simulink model "V2021_M2_P1_P"  (R2021a)
settings: Solver=VariableStepAuto  StartTime=0.0  StopTime=500  RelTol=1e-3
undefined symbols (not defined in the file): f_eff, J_eff, Kb, Ktn, L, Pos_ref, R, time
settings Model: Creator=azzam  LastModifiedBy=azzam
settings DebuggingCC: UnconnectedInputMsg=none  UnconnectedOutputMsg=none  UnconnectedLineMsg=none
settings ModelReferenceCC: EnableRefExpFcnMdlSchedulingChecks=off
settings RTWCC: Description=Generic Real-Time Target  DLArmComputeVersion=20.02.1

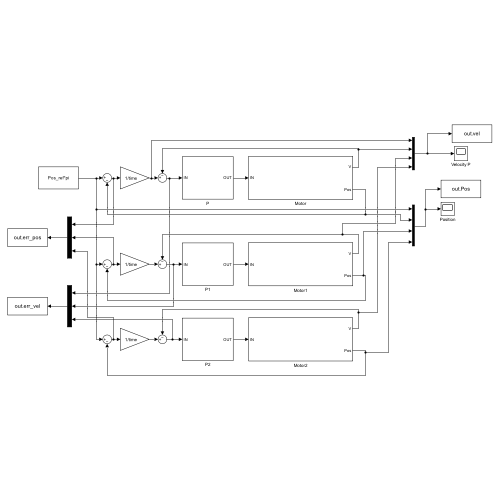
[thumbnail: Simulink's stored preview of the top-level diagram]
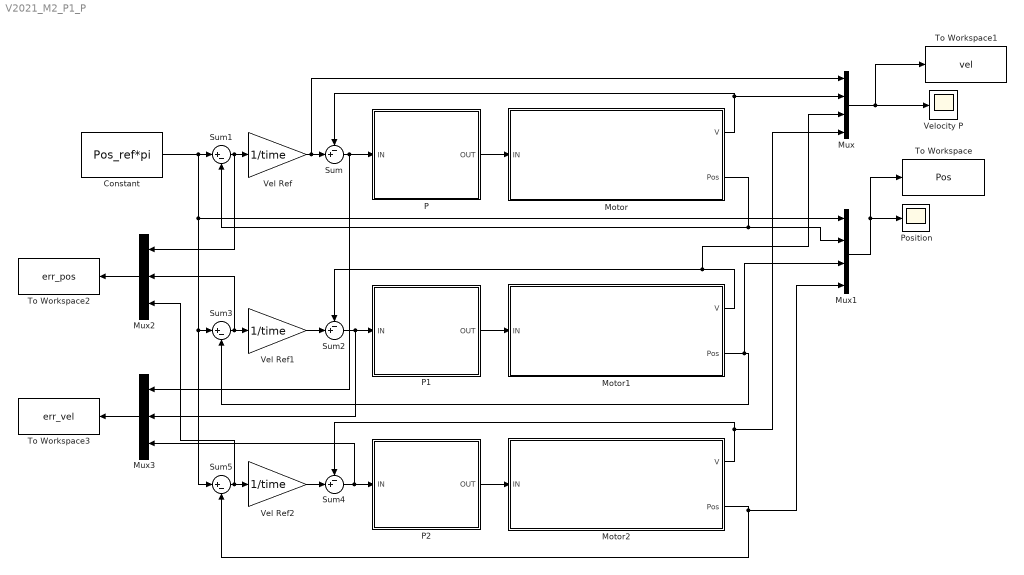
== system V2021_M2_P1_P ==
  Constant : Constant  Value=Pos_ref*pi
  Motor : Subsystem
  Motor1 : Subsystem
  Motor2 : Subsystem
  Mux : Mux
  Mux1 : Mux
  Mux2 : Mux  Inputs=3
  Mux3 : Mux  Inputs=3
  P : Subsystem
  P1 : Subsystem
  P2 : Subsystem
  Position : Scope
  Sum : Sum  Inputs=-+|
  Sum1 : Sum  Inputs=|+-
  Sum2 : Sum  Inputs=-+|
  Sum3 : Sum  Inputs=|+-
  Sum4 : Sum  Inputs=-+|
  Sum5 : Sum  Inputs=|+-
  To Workspace : ToWorkspace  VariableName=Pos  SaveFormat=Timeseries  SampleTime=-1
  To Workspace1 : ToWorkspace  VariableName=vel  SaveFormat=Timeseries  SampleTime=-1
  To Workspace2 : ToWorkspace  VariableName=err_pos  SaveFormat=Timeseries  SampleTime=-1
  To Workspace3 : ToWorkspace  VariableName=err_vel  SaveFormat=Timeseries  SampleTime=-1
  Vel Ref : Gain  Gain=1/time
  Vel Ref1 : Gain  Gain=1/time
  Vel Ref2 : Gain  Gain=1/time
  Velocity P : Scope
  wires:
  Sum/1 -> P/1(IN), Mux3/1
  Sum1/1 -> Mux2/1, Vel Ref/1
  Vel Ref/1 -> Sum/2, Mux/1
  Motor/2(Pos) -> Sum1/2, Mux1/2
  Mux/1 -> To Workspace1/1, Velocity P/1
  Motor/1(V) -> Sum/1, Mux/2
  P/1(OUT) -> Motor/1(IN)
  Mux1/1 -> To Workspace/1, Position/1
  Motor1/2(Pos) -> Mux1/3, Sum3/2
  P1/1(OUT) -> Motor1/1(IN)
  Motor1/1(V) -> Mux/3, Sum2/1
  Sum3/1 -> Mux2/2, Vel Ref1/1
  Sum2/1 -> P1/1(IN), Mux3/2
  Vel Ref1/1 -> Sum2/2
  Constant/1 -> Sum5/1, Sum3/1, Mux1/1, Sum1/1
  Vel Ref2/1 -> Sum4/2
  Motor2/1(V) -> Mux/4, Sum4/1
  Sum4/1 -> P2/1(IN), Mux3/3
  Sum5/1 -> Mux2/3, Vel Ref2/1
  P2/1(OUT) -> Motor2/1(IN)
  Motor2/2(Pos) -> Mux1/4, Sum5/2
  Mux2/1 -> To Workspace2/1
  Mux3/1 -> To Workspace3/1

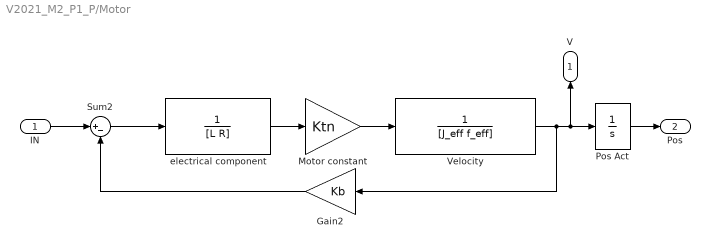
== system V2021_M2_P1_P/Motor ==
  IN : Inport
  Gain2 : Gain  Gain=Kb
  Motor constant : Gain  Gain=Ktn
  Pos Act : Integrator
  Sum2 : Sum  Inputs=|+-
  Velocity : TransferFcn  Denominator=[J_eff f_eff]
  electrical component : TransferFcn  Denominator=[L R]
  V : Outport
  Pos : Outport  Port=2
  wires:
  electrical component/1 -> Motor constant/1
  Motor constant/1 -> Velocity/1
  Sum2/1 -> electrical component/1
  IN/1 -> Sum2/1
  Gain2/1 -> Sum2/2
  Velocity/1 -> V/1, Pos Act/1, Gain2/1
  Pos Act/1 -> Pos/1

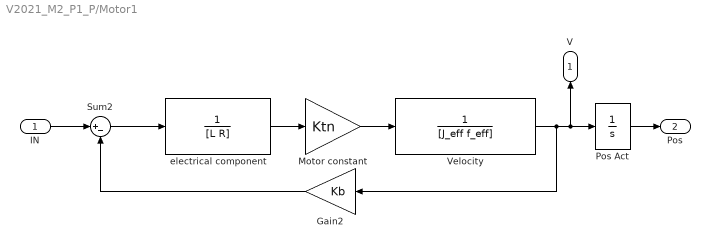
== system V2021_M2_P1_P/Motor1 ==
  IN : Inport
  Gain2 : Gain  Gain=Kb
  Motor constant : Gain  Gain=Ktn
  Pos Act : Integrator
  Sum2 : Sum  Inputs=|+-
  Velocity : TransferFcn  Denominator=[J_eff f_eff]
  electrical component : TransferFcn  Denominator=[L R]
  V : Outport
  Pos : Outport  Port=2
  wires:
  electrical component/1 -> Motor constant/1
  Motor constant/1 -> Velocity/1
  Sum2/1 -> electrical component/1
  IN/1 -> Sum2/1
  Gain2/1 -> Sum2/2
  Velocity/1 -> V/1, Pos Act/1, Gain2/1
  Pos Act/1 -> Pos/1

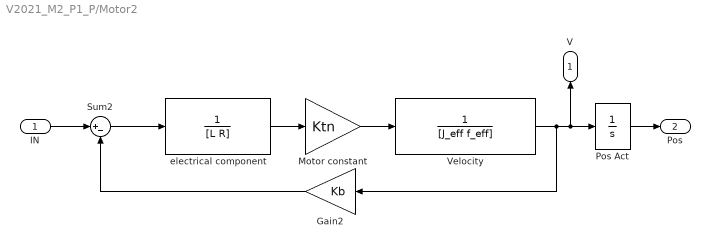
== system V2021_M2_P1_P/Motor2 ==
  IN : Inport
  Gain2 : Gain  Gain=Kb
  Motor constant : Gain  Gain=Ktn
  Pos Act : Integrator
  Sum2 : Sum  Inputs=|+-
  Velocity : TransferFcn  Denominator=[J_eff f_eff]
  electrical component : TransferFcn  Denominator=[L R]
  V : Outport
  Pos : Outport  Port=2
  wires:
  electrical component/1 -> Motor constant/1
  Motor constant/1 -> Velocity/1
  Sum2/1 -> electrical component/1
  IN/1 -> Sum2/1
  Gain2/1 -> Sum2/2
  Velocity/1 -> V/1, Pos Act/1, Gain2/1
  Pos Act/1 -> Pos/1

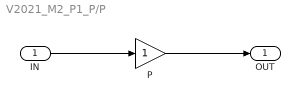
== system V2021_M2_P1_P/P ==
  IN : Inport
  P : Gain
  OUT : Outport
  wires:
  IN/1 -> P/1
  P/1 -> OUT/1

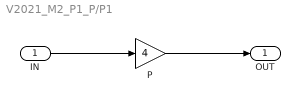
== system V2021_M2_P1_P/P1 ==
  IN : Inport
  P : Gain  Gain=4
  OUT : Outport
  wires:
  P/1 -> OUT/1
  IN/1 -> P/1

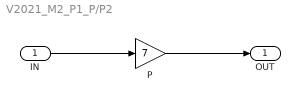
== system V2021_M2_P1_P/P2 ==
  IN : Inport
  P : Gain  Gain=7
  OUT : Outport
  wires:
  P/1 -> OUT/1
  IN/1 -> P/1
